simulink model "Test_Encoder"  (R2023b)
settings: Solver=VariableStepAuto  StartTime=0.0  StopTime=10.0  RelTol=1e-3
libraries: arduinosensorlib x2
settings Model: Creator=marqu  LastModifiedBy=marqu

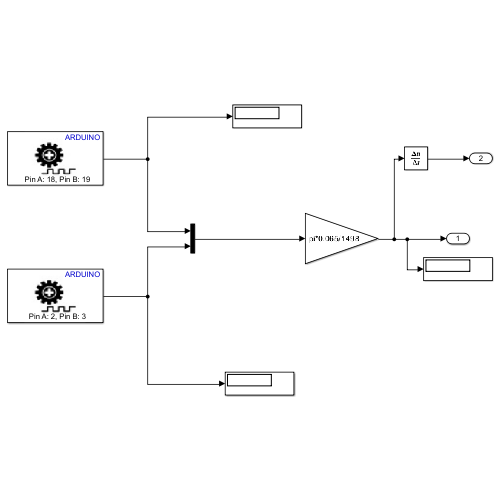
[thumbnail: Simulink's stored preview of the top-level diagram]
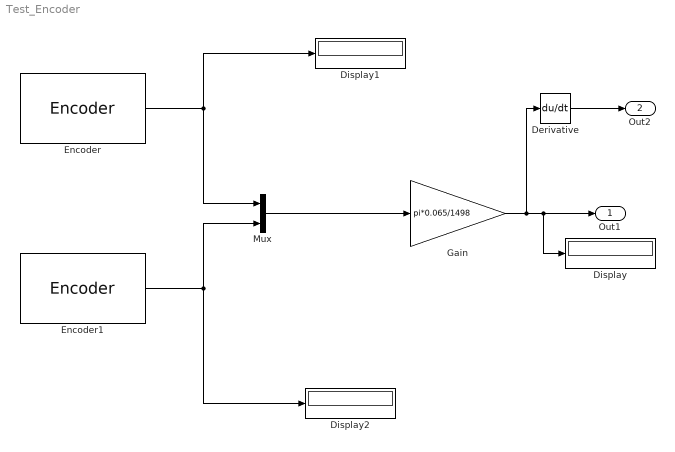
== system Test_Encoder ==
  Derivative : Derivative
  Display : Display
  Display1 : Display
  Display2 : Display
  Encoder : arduinosensorlib/Encoder  InputA=18  InputB=19  Mode=No reset  SampleTime=0.1
  Encoder1 : arduinosensorlib/Encoder  InputA=2  InputB=3  Mode=No reset  SampleTime=0.1
  Gain : Gain  Gain=pi*0.065/1498
  Mux : Mux  Inputs=2
  Out1 : Outport
  Out2 : Outport  Port=2
  wires:
  Encoder/1 -> Mux/1, Display1/1
  Encoder1/1 -> Display2/1, Mux/2
  Mux/1 -> Gain/1
  Gain/1 -> Derivative/1, Display/1, Out1/1
  Derivative/1 -> Out2/1
